simulink model "basic_serial_read"  (R2021a)
settings: Solver=FixedStepDiscrete  StartTime=0.0  StopTime=5  FixedStep=1/50  RelTol=1e-3
undefined symbols (not defined in the file): CR, LF
libraries: instrumentseriallib x2
settings Model: Creator=bruders  LastModifiedBy=steve
settings DataIOCC: ReturnWorkspaceOutputs=off

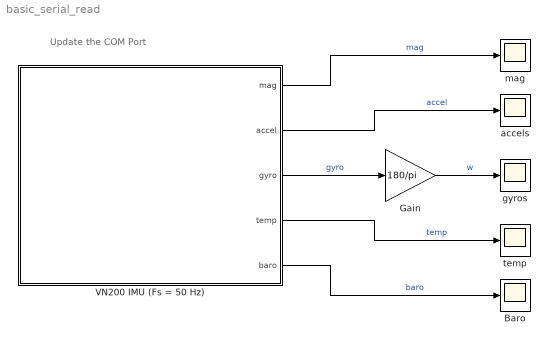
== system basic_serial_read ==
  note: Update the COM Port
  Baro : Scope
  Gain : Gain  Gain=180/pi
  VN200 IMU (Fs = 50 Hz) : Subsystem
      mask Display: image('$imagefile'); % Use "Edit Image" on toolstrip to change.
  accels : Scope
  gyros : Scope
  mag : Scope
  temp : Scope
  wires:
  Gain/1 -> gyros/1  "w"
  VN200 IMU (Fs = 50 Hz)/1(mag) -> mag/1  "mag"
  VN200 IMU (Fs = 50 Hz)/2(accel) -> accels/1  "accel"
  VN200 IMU (Fs = 50 Hz)/3(gyro) -> Gain/1  "gyro"
  VN200 IMU (Fs = 50 Hz)/4(temp) -> temp/1  "temp"
  VN200 IMU (Fs = 50 Hz)/5(baro) -> Baro/1  "baro"

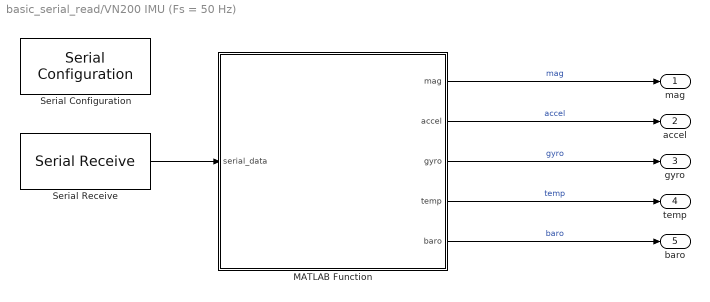
== system basic_serial_read/VN200 IMU (Fs = 50 Hz) ==
  MATLAB Function : MATLAB Function  TreatAsAtomicUnit=on
  Serial Configuration : instrumentseriallib/Serial Configuration  Priority=-200000  Port=<Select a port...>  ComPort=<Select a port...>  BaudRate=115200  DataBits=8  Parity=none  StopBits=1  ByteOrder=little-endian  FlowControl=none  Timeout=10  SimulateUsing=Interpreted execution  BlockInModel=on
  Serial Receive : instrumentseriallib/Serial Receive  Priority=1  Port=<Select a port...>  ComPort=<Select a port...>  DataType=uint8  SaveDataType=uint8  ToggleHeader=on  Header='$VNIMU,'  ToggleTerminator=on  Terminator=CR/LF ('\r\n')  CustomTerminator=[]  ToggleDataSize=on  DataSize=[1 101]  EnableBlockingMode=on  ActionDataUnavailable=Error  ActionWhenDataUnavailable=Error  CustomValue=0  SampleTime=0.02  SimulateUsing=Interpreted execution  BlockInModel=on
  mag : Outport
  accel : Outport  Port=2
  gyro : Outport  Port=3
  temp : Outport  Port=4
  baro : Outport  Port=5
  wires:
  Serial Receive/1 -> MATLAB Function/1(serial_data)
  MATLAB Function/4(temp) -> temp/1  "temp"
  MATLAB Function/1(mag) -> mag/1  "mag"
  MATLAB Function/3(gyro) -> gyro/1  "gyro"
  MATLAB Function/2(accel) -> accel/1  "accel"
  MATLAB Function/5(baro) -> baro/1  "baro"

== matlab function basic_serial_read/VN200 IMU (Fs = 50 Hz)/MATLAB Function ==
  data: serial_data input; mag output double; accel output double; gyro output double; temp output double; baro output double
function [mag, accel, gyro, temp, baro] = extract_imu_sigs(serial_data)
% Description:
%   This function reads data from the VN200 IMU at 50 Hz
%
% Input:
%   serial_data - ASCII data from the serial port (char array UTF8)
%
% Output:
%   mag     - Magnetometer output as a 3x1 array (in Gauss)
%   accel   - Accelerometer output as a 3x1 array (in m/s^2)
%   gyro    - Gyro output as a 3x1 array (in rad/s)
%   temp    - IMU temperature as a scalar (in °C)
%   baro    - Barometer output as a scalar (in kPa)
%
% NOTES:
%   The VN200 was configured to output the '$VNIMU' stream at 50 Hz on startup

    % Convert ASCII character array to a string.  Example of the IMU data string:
    % $VNIMU,-00.0350,+00.4222,-00.6643,-00.015,+00.019,+09.948,+00.002066,-00.008442,-00.044656,+20.7,+084.322*66
    %       ,   Magnetomrter data      ,     Accel data        ,           Gyro       data      , Temp , baro
    % The last three bytes are checksum
    sigs = char(serial_data);      

    % Convert the Magnetometer portion of the string to floating point
    mag  = real([str2double(sigs(1:8))      % (Gauss)
            str2double(sigs(10:17))
            str2double(sigs(19:26))]);

    % Convert the Accelerometer portion of the string to floating point
    accel = real([str2double(sigs(28:34))   % (m/s^2)
             str2double(sigs(36:42))
             str2double(sigs(44:50))]);

    % Convert the Gyro portion of the string to floating point     
    gyro = real([str2double(sigs(52:61))    % (rad/s)
            str2double(sigs(63:72))
            str2double(sigs(74:83))]);

    % Convert the temperature portion of the string to floating point         
    temp  = real(str2double(sigs(85:89)));  % (°C)

    % Convert the Barometer portion of the string to floating point
    baro  = real(str2double(sigs(91:98)));  % (kPa)

    % A simple check of the integrity of the string (not checksum)
    if sigs(99) ~= '*'
        error('Data is bad');
    end
end     % End of function
